simulink model "Enum"  (R2016b)
settings: Solver=FixedStepDiscrete  StartTime=0.0  StopTime=10.0  RelTol=1e-3
undefined symbols (not defined in the file or in its folder): BasicColors
libraries: simulink x1
settings Model: Creator=3essawy  LastModifiedBy=3essawy
settings OptimizationCC: DefaultParameterBehavior=Inlined
settings DebuggingCC: ParameterTunabilityLossMsg=error
settings RTWCC: SystemTargetFile=ert.tlc  GenCodeOnly=on  TemplateMakefile=ert_default_tmf  Description=Embedded Coder  GenerateReport=on  IncludeHyperlinkInReport=on  LaunchReport=on  GenerateTraceInfo=on  GenerateTraceReport=on  GenerateTraceReportSl=on  GenerateTraceReportSf=on  GenerateTraceReportEml=on
settings CodeAppCC: ForceParamTrailComments=on  IgnoreCustomStorageClasses=off  OperatorAnnotations=on  SimulinkDataObjDesc=on  SFDataObjDesc=on  MATLABFcnDesc=on  InsertBlockDesc=on  MATLABSourceComments=on
settings ERTTargetCC: TargetLangStandard=C99 (ISO)  GenerateSampleERTMain=on  InlinedParameterPlacement=NonHierarchical  ERTCustomFileTemplate=example_file_process.tlc  EnableUserReplacementTypes=on

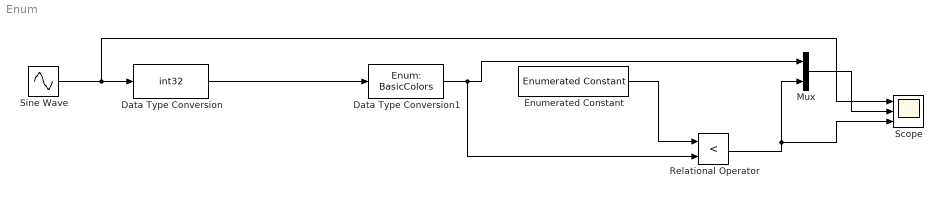
== system Enum ==
  Data Type Conversion : DataTypeConversion  OutDataTypeStr=int32
  Data Type Conversion1 : DataTypeConversion  OutDataTypeStr=Enum: BasicColors
  Enumerated Constant : simulink/Sources/Enumerated Constant  OutDataTypeStr=Enum: BasicColors  Value=BasicColors.Yellow  SampleTime=inf
  Mux : Mux  Inputs=2
  Relational Operator : RelationalOperator  Operator=<  OutDataTypeStr=BasicColors  RndMeth=Simplest
  Scope : Scope  NumInputPorts=3
  Sine Wave : Sin  SineType=Sample based  SampleTime=1
  wires:
  Data Type Conversion/1 -> Data Type Conversion1/1
  Sine Wave/1 -> Scope/1, Data Type Conversion/1
  Enumerated Constant/1 -> Relational Operator/1
  Relational Operator/1 -> Mux/2, Scope/3
  Data Type Conversion1/1 -> Mux/1, Relational Operator/2
  Mux/1 -> Scope/2
